simulink model "V2x_blockset"  (Simulink 7.6)
settings: Solver=ode45  StartTime=0.0  StopTime=10.0  RelTol=1e-3
undefined symbols (not defined in the file or in its folder): intmax, Newton, Raphson
libraries: simulink x53
(part 1 of 3)
settings Model: Creator=MarcinB  LastModifiedBy=pastora
settings SFSimCC: SimParseCustomCode=off

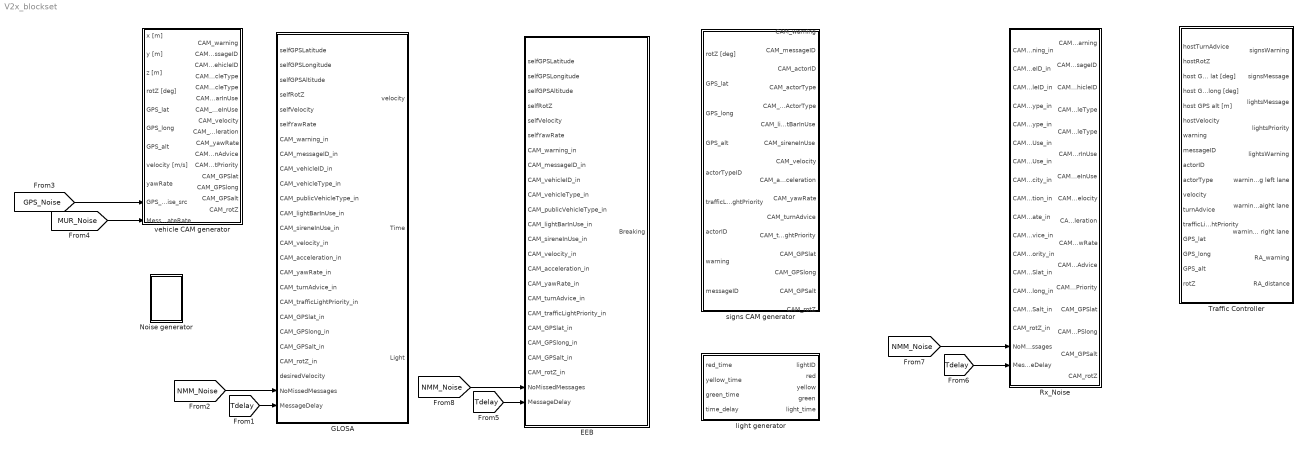
== system V2x_blockset ==
  EEB : Subsystem
  GLOSA : Subsystem
  Noise generator : Subsystem
  Rx_Noise : Subsystem
  Traffic Controller : Subsystem
  light generator : Subsystem
  signs CAM generator : Subsystem
  vehicle CAM generator : Subsystem
  wires:
  [NMM_Noise] -> GLOSA/24(NoMissedMessages)
  [Tdelay] -> GLOSA/25(MessageDelay)
  [MUR_Noise] -> vehicle CAM generator/11(MessageUpdateRate)
  [GPS_Noise] -> vehicle CAM generator/10(GPS_Noise_src)
  [NMM_Noise] -> Rx_Noise/17(NoMissedMessages)
  [Tdelay] -> Rx_Noise/18(MessageDelay)
  [NMM_Noise] -> EEB/23(NoMissedMessages)
  [Tdelay] -> EEB/24(MessageDelay)

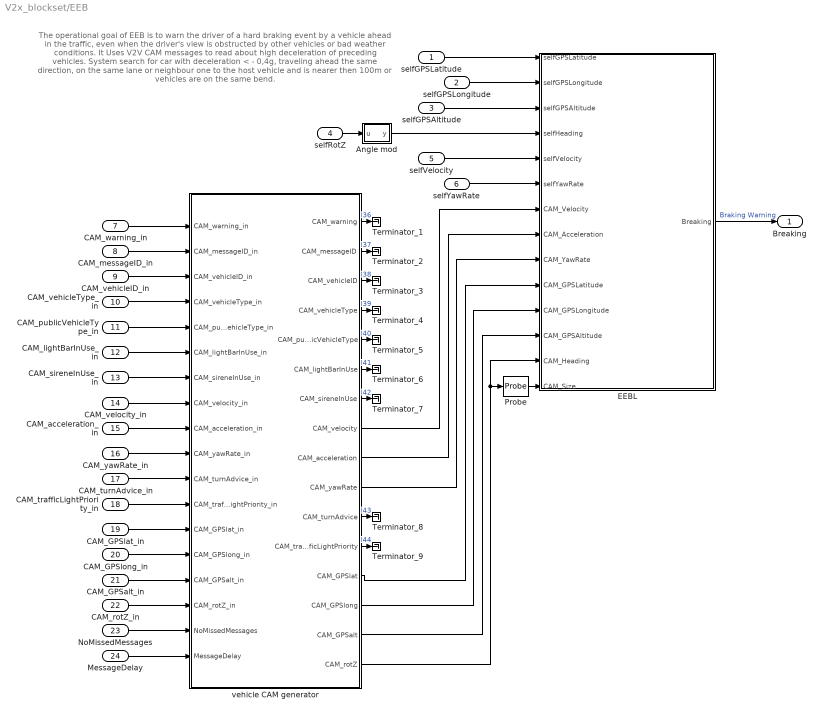
== system V2x_blockset/EEB ==
  note: The operational goal of EEB is to warn the driver of
      | a hard braking event by a vehicle ahead in the traffic,
      |  even when the driver's view is obstructed by
      |  other vehicles or bad weather conditions. It Uses V2V CAM
      | messages to read about high deceleration of preceding vehicles.
      | System search for car with deceleration < - 0,4g, traveling ahead
      |  the same direction, on the same lane or neighbour one to the host
      |  vehicle and is nearer then 100m or vehicles are on the same bend.
  selfGPSLatitude : Inport
  selfGPSLongitude : Inport  Port=2
  selfGPSAltitude : Inport  Port=3
  selfRotZ : Inport  Port=4
  selfVelocity : Inport  Port=5
  selfYawRate : Inport  Port=6
  CAM_warning_in : Inport  Port=7
  CAM_messageID_in : Inport  Port=8
  CAM_vehicleID_in : Inport  Port=9
  CAM_vehicleType_in : Inport  Port=10
  CAM_publicVehicleType_in : Inport  Port=11
  CAM_lightBarInUse_in : Inport  Port=12
  CAM_sireneInUse_in : Inport  Port=13
  CAM_velocity_in : Inport  Port=14
  CAM_acceleration_in : Inport  Port=15
  CAM_yawRate_in : Inport  Port=16
  CAM_turnAdvice_in : Inport  Port=17
  CAM_trafficLightPriority_in : Inport  Port=18
  CAM_GPSlat_in : Inport  Port=19
  CAM_GPSlong_in : Inport  Port=20
  CAM_GPSalt_in : Inport  Port=21
  CAM_rotZ_in : Inport  Port=22
  NoMissedMessages : Inport  Port=23
  MessageDelay : Inport  Port=24
  Angle mod : Stateflow chart  TreatAsAtomicUnit=on
  EEBL : Stateflow chart  TreatAsAtomicUnit=on
  Probe : Probe  ProbeWidth=off  ProbeSampleTime=off  ProbeComplexSignal=off  ProbeSignalDimensions=on
  Terminator_{1..9} (9 alike) : Terminator
  vehicle CAM generator : Subsystem
  Breaking : Outport
  wires:
  CAM_warning_in/1 -> vehicle CAM generator/1(CAM_warning_in)
  CAM_messageID_in/1 -> vehicle CAM generator/2(CAM_messageID_in)
  CAM_vehicleID_in/1 -> vehicle CAM generator/3(CAM_vehicleID_in)
  CAM_vehicleType_in/1 -> vehicle CAM generator/4(CAM_vehicleType_in)
  CAM_publicVehicleType_in/1 -> vehicle CAM generator/5(CAM_publicVehicleType_in)
  CAM_lightBarInUse_in/1 -> vehicle CAM generator/6(CAM_lightBarInUse_in)
  CAM_sireneInUse_in/1 -> vehicle CAM generator/7(CAM_sireneInUse_in)
  CAM_velocity_in/1 -> vehicle CAM generator/8(CAM_velocity_in)
  CAM_acceleration_in/1 -> vehicle CAM generator/9(CAM_acceleration_in)
  CAM_yawRate_in/1 -> vehicle CAM generator/10(CAM_yawRate_in)
  CAM_turnAdvice_in/1 -> vehicle CAM generator/11(CAM_turnAdvice_in)
  CAM_trafficLightPriority_in/1 -> vehicle CAM generator/12(CAM_trafficLightPriority_in)
  CAM_GPSlat_in/1 -> vehicle CAM generator/13(CAM_GPSlat_in)
  CAM_GPSlong_in/1 -> vehicle CAM generator/14(CAM_GPSlong_in)
  CAM_GPSalt_in/1 -> vehicle CAM generator/15(CAM_GPSalt_in)
  CAM_rotZ_in/1 -> vehicle CAM generator/16(CAM_rotZ_in)
  EEBL/1(Breaking) -> Breaking/1  "Braking Warning"
  selfGPSLatitude/1 -> EEBL/1(selfGPSLatitude)
  selfGPSLongitude/1 -> EEBL/2(selfGPSLongitude)
  selfGPSAltitude/1 -> EEBL/3(selfGPSAltitude)
  selfRotZ/1 -> Angle mod/1(u)
  selfVelocity/1 -> EEBL/5(selfVelocity)
  selfYawRate/1 -> EEBL/6(selfYawRate)
  NoMissedMessages/1 -> vehicle CAM generator/17(NoMissedMessages)
  MessageDelay/1 -> vehicle CAM generator/18(MessageDelay)
  vehicle CAM generator/8(CAM_velocity) -> EEBL/7(CAM_Velocity)
  vehicle CAM generator/16(CAM_rotZ) -> EEBL/13(CAM_Heading), Probe/1
  vehicle CAM generator/13(CAM_GPSlat) -> EEBL/10(CAM_GPSLatitude)
  vehicle CAM generator/14(CAM_GPSlong) -> EEBL/11(CAM_GPSLongitude)
  vehicle CAM generator/15(CAM_GPSalt) -> EEBL/12(CAM_GPSAltitude)
  vehicle CAM generator/10(CAM_yawRate) -> EEBL/9(CAM_YawRate)
  vehicle CAM generator/9(CAM_acceleration) -> EEBL/8(CAM_Acceleration)
  Angle mod/1(y) -> EEBL/4(selfHeading)
  Probe/1 -> EEBL/14(CAM_Size)
  vehicle CAM generator/1(CAM_warning) -> Terminator_1/1  "l36"
  vehicle CAM generator/2(CAM_messageID) -> Terminator_2/1  "l37"
  vehicle CAM generator/3(CAM_vehicleID) -> Terminator_3/1  "l38"
  vehicle CAM generator/4(CAM_vehicleType) -> Terminator_4/1  "l39"
  vehicle CAM generator/5(CAM_publicVehicleType) -> Terminator_5/1  "l40"
  vehicle CAM generator/6(CAM_lightBarInUse) -> Terminator_6/1  "l41"
  vehicle CAM generator/7(CAM_sireneInUse) -> Terminator_7/1  "l42"
  vehicle CAM generator/11(CAM_turnAdvice) -> Terminator_8/1  "l43"
  vehicle CAM generator/12(CAM_trafficLightPriority) -> Terminator_9/1  "l44"

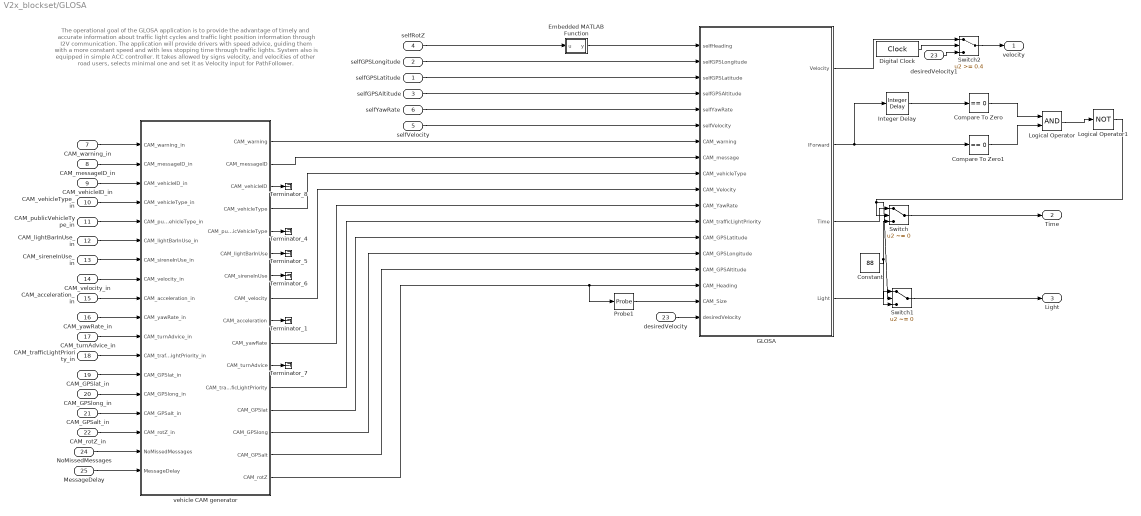
== system V2x_blockset/GLOSA ==
  note: The operational goal of the GLOSA application is to provide the advantage of
      |  timely and accurate information about traffic light cycles and
      |  traffic light position information through I2V communication.
      |  The application will provide drivers with speed advice, guiding them
      |  with a more constant speed and with less stopping time through traffic lights.
      |  System also is equipped in simple ACC controller.
      | It takes allowed by signs velocity, and velocities of other road users,
      |  selects minimal one and set it as Velocity input for PathFollower.
  selfGPSLatitude : Inport
  selfGPSLongitude : Inport  Port=2
  selfGPSAltitude : Inport  Port=3
  selfRotZ : Inport  Port=4
  selfVelocity : Inport  Port=5
  selfYawRate : Inport  Port=6
  CAM_warning_in : Inport  Port=7
  CAM_messageID_in : Inport  Port=8
  CAM_vehicleID_in : Inport  Port=9
  CAM_vehicleType_in : Inport  Port=10
  CAM_publicVehicleType_in : Inport  Port=11
  CAM_lightBarInUse_in : Inport  Port=12
  CAM_sireneInUse_in : Inport  Port=13
  CAM_velocity_in : Inport  Port=14
  CAM_acceleration_in : Inport  Port=15
  CAM_yawRate_in : Inport  Port=16
  CAM_turnAdvice_in : Inport  Port=17
  CAM_trafficLightPriority_in : Inport  Port=18
  CAM_GPSlat_in : Inport  Port=19
  CAM_GPSlong_in : Inport  Port=20
  CAM_GPSalt_in : Inport  Port=21
  CAM_rotZ_in : Inport  Port=22
  desiredVelocity : Inport  Port=23
  NoMissedMessages : Inport  Port=24
  MessageDelay : Inport  Port=25
  Compare To Zero : simulink/Logic and Bit Operations/Compare To Zero  SystemSampleTime=-1  relop===  LogicOutDataTypeMode=boolean
  Compare To Zero1 : simulink/Logic and Bit Operations/Compare To Zero  SystemSampleTime=-1  relop===  LogicOutDataTypeMode=boolean
  Constant : Constant  Value=88
  Digital Clock : DigitalClock
  Embedded MATLAB Function : Stateflow chart  TreatAsAtomicUnit=on
  GLOSA : Stateflow chart  TreatAsAtomicUnit=on
  Integer Delay : simulink/Discrete/Integer Delay  vinit=0.0  samptime=-1  NumDelays=5
  Logical Operator : Logic  AllPortsSameDT=off  OutDataTypeStr=boolean
  Logical Operator1 : Logic  Operator=NOT  AllPortsSameDT=off  OutDataTypeStr=boolean
  Probe1 : Probe  ProbeWidth=off  ProbeSampleTime=off  ProbeComplexSignal=off  ProbeSignalDimensions=on
  Switch : Switch  Criteria=u2 ~= 0
  Switch1 : Switch  Criteria=u2 ~= 0
  Switch2 : Switch  Threshold=0.4
  Terminator_{1,4..8} (6 alike) : Terminator
  desiredVelocity1 : InportShadow  Port=23
  vehicle CAM generator : Subsystem
  velocity : Outport
  Time : Outport  Port=2
  Light : Outport  Port=3
  wires:
  vehicle CAM generator/10(CAM_yawRate) -> GLOSA/11(CAM_YawRate)
  vehicle CAM generator/16(CAM_rotZ) -> GLOSA/16(CAM_Heading), Probe1/1
  vehicle CAM generator/15(CAM_GPSalt) -> GLOSA/15(CAM_GPSAltitude)
  vehicle CAM generator/13(CAM_GPSlat) -> GLOSA/13(CAM_GPSLatitude)
  vehicle CAM generator/14(CAM_GPSlong) -> GLOSA/14(CAM_GPSLongitude)
  vehicle CAM generator/8(CAM_velocity) -> GLOSA/10(CAM_Velocity)
  selfGPSLatitude/1 -> GLOSA/3(selfGPSLatitude)
  selfGPSLongitude/1 -> GLOSA/2(selfGPSLongitude)
  selfGPSAltitude/1 -> GLOSA/4(selfGPSAltitude)
  selfRotZ/1 -> Embedded MATLAB Function/1(u)
  selfVelocity/1 -> GLOSA/6(selfVelocity)
  selfYawRate/1 -> GLOSA/5(selfYawRate)
  CAM_warning_in/1 -> vehicle CAM generator/1(CAM_warning_in)
  CAM_messageID_in/1 -> vehicle CAM generator/2(CAM_messageID_in)
  CAM_vehicleID_in/1 -> vehicle CAM generator/3(CAM_vehicleID_in)
  CAM_vehicleType_in/1 -> vehicle CAM generator/4(CAM_vehicleType_in)
  CAM_publicVehicleType_in/1 -> vehicle CAM generator/5(CAM_publicVehicleType_in)
  CAM_lightBarInUse_in/1 -> vehicle CAM generator/6(CAM_lightBarInUse_in)
  CAM_sireneInUse_in/1 -> vehicle CAM generator/7(CAM_sireneInUse_in)
  CAM_velocity_in/1 -> vehicle CAM generator/8(CAM_velocity_in)
  CAM_acceleration_in/1 -> vehicle CAM generator/9(CAM_acceleration_in)
  CAM_yawRate_in/1 -> vehicle CAM generator/10(CAM_yawRate_in)
  CAM_turnAdvice_in/1 -> vehicle CAM generator/11(CAM_turnAdvice_in)
  CAM_trafficLightPriority_in/1 -> vehicle CAM generator/12(CAM_trafficLightPriority_in)
  CAM_GPSlat_in/1 -> vehicle CAM generator/13(CAM_GPSlat_in)
  CAM_GPSlong_in/1 -> vehicle CAM generator/14(CAM_GPSlong_in)
  CAM_GPSalt_in/1 -> vehicle CAM generator/15(CAM_GPSalt_in)
  CAM_rotZ_in/1 -> vehicle CAM generator/16(CAM_rotZ_in)
  vehicle CAM generator/1(CAM_warning) -> GLOSA/7(CAM_warning)
  vehicle CAM generator/2(CAM_messageID) -> GLOSA/8(CAM_message)
  vehicle CAM generator/4(CAM_vehicleType) -> GLOSA/9(CAM_vehicleType)
  vehicle CAM generator/5(CAM_publicVehicleType) -> Terminator_4/1
  vehicle CAM generator/6(CAM_lightBarInUse) -> Terminator_5/1
  vehicle CAM generator/7(CAM_sireneInUse) -> Terminator_6/1
  vehicle CAM generator/11(CAM_turnAdvice) -> Terminator_7/1
  vehicle CAM generator/12(CAM_trafficLightPriority) -> GLOSA/12(CAM_trafficLightPriority)
  desiredVelocity/1 -> GLOSA/18(desiredVelocity)
  vehicle CAM generator/3(CAM_vehicleID) -> Terminator_8/1
  Embedded MATLAB Function/1(y) -> GLOSA/1(selfHeading)
  NoMissedMessages/1 -> vehicle CAM generator/17(NoMissedMessages)
  MessageDelay/1 -> vehicle CAM generator/18(MessageDelay)
  Probe1/1 -> GLOSA/17(CAM_Size)
  vehicle CAM generator/9(CAM_acceleration) -> Terminator_1/1
  GLOSA/3(Time) -> Switch/1
  GLOSA/4(Light) -> Switch1/1
  GLOSA/2(lForward) -> Integer Delay/1, Compare To Zero1/1
  Constant/1 -> Switch/3, Switch1/3
  Switch1/1 -> Light/1
  Switch/1 -> Time/1
  Integer Delay/1 -> Compare To Zero/1
  Compare To Zero/1 -> Logical Operator/1
  Compare To Zero1/1 -> Logical Operator/2
  Logical Operator/1 -> Logical Operator1/1
  Logical Operator1/1 -> Switch/2, Switch1/2
  Digital Clock/1 -> Switch2/2
  Switch2/1 -> velocity/1
  GLOSA/1(Velocity) -> Switch2/1
  desiredVelocity1/1 -> Switch2/3

== system V2x_blockset/Noise generator ==
  DISPLAY : M-S-Function  FunctionName=msfcn_V2X_PlotSpeed
  Scope1 : Scope  NumInputPorts=4
      settings: YMin=-5~-5~-5~-5  YMax=5~5~5~5
  tag scope: GPS_Noise=global, MUR_Noise=global, NMM_Noise=global, Tdelay=global
  wires:
  DISPLAY/1 -> Scope1/1, [GPS_Noise]
  DISPLAY/2 -> Scope1/2, [MUR_Noise]
  DISPLAY/3 -> Scope1/3, [NMM_Noise]
  DISPLAY/4 -> Scope1/4, [Tdelay]

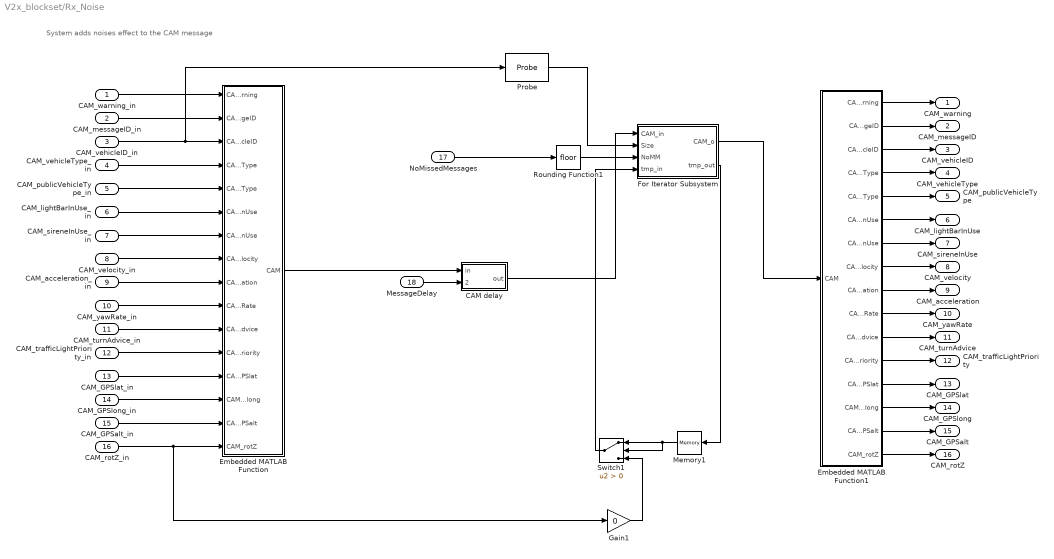
== system V2x_blockset/Rx_Noise ==
  note: System adds noises effect to the CAM message
  CAM_warning_in : Inport
  CAM_messageID_in : Inport  Port=2
  CAM_vehicleID_in : Inport  Port=3
  CAM_vehicleType_in : Inport  Port=4
  CAM_publicVehicleType_in : Inport  Port=5
  CAM_lightBarInUse_in : Inport  Port=6
  CAM_sireneInUse_in : Inport  Port=7
  CAM_velocity_in : Inport  Port=8
  CAM_acceleration_in : Inport  Port=9
  CAM_yawRate_in : Inport  Port=10
  CAM_turnAdvice_in : Inport  Port=11
  CAM_trafficLightPriority_in : Inport  Port=12
  CAM_GPSlat_in : Inport  Port=13
  CAM_GPSlong_in : Inport  Port=14
  CAM_GPSalt_in : Inport  Port=15
  CAM_rotZ_in : Inport  Port=16
  NoMissedMessages : Inport  Port=17
  MessageDelay : Inport  Port=18
  CAM delay : Subsystem
  Embedded MATLAB Function : Stateflow chart  TreatAsAtomicUnit=on
  Embedded MATLAB Function1 : Stateflow chart  TreatAsAtomicUnit=on
  For Iterator Subsystem : Subsystem  TreatAsAtomicUnit=on
  Gain1 : Gain  Gain=0
  Memory1 : Memory
  Probe : Probe  ProbeWidth=off  ProbeSampleTime=off  ProbeComplexSignal=off  ProbeSignalDimensions=on
  Rounding Function1 : Rounding
  Switch1 : Switch  Criteria=u2 > Threshold
  CAM_warning : Outport
  CAM_messageID : Outport  Port=2
  CAM_vehicleID : Outport  Port=3
  CAM_vehicleType : Outport  Port=4
  CAM_publicVehicleType : Outport  Port=5
  CAM_lightBarInUse : Outport  Port=6
  CAM_sireneInUse : Outport  Port=7
  CAM_velocity : Outport  Port=8
  CAM_acceleration : Outport  Port=9
  CAM_yawRate : Outport  Port=10
  CAM_turnAdvice : Outport  Port=11
  CAM_trafficLightPriority : Outport  Port=12
  CAM_GPSlat : Outport  Port=13
  CAM_GPSlong : Outport  Port=14
  CAM_GPSalt : Outport  Port=15
  CAM_rotZ : Outport  Port=16
  wires:
  Embedded MATLAB Function1/16(CAM_rotZ) -> CAM_rotZ/1
  Embedded MATLAB Function1/15(CAM_GPSalt) -> CAM_GPSalt/1
  Embedded MATLAB Function1/14(CAM_GPSlong) -> CAM_GPSlong/1
  Embedded MATLAB Function1/13(CAM_GPSlat) -> CAM_GPSlat/1
  Embedded MATLAB Function1/12(CAM_trafficLightPriority) -> CAM_trafficLightPriority/1
  Embedded MATLAB Function1/11(CAM_turnAdvice) -> CAM_turnAdvice/1
  Embedded MATLAB Function1/10(CAM_yawRate) -> CAM_yawRate/1
  Embedded MATLAB Function1/9(CAM_acceleration) -> CAM_acceleration/1
  Embedded MATLAB Function1/8(CAM_velocity) -> CAM_velocity/1
  Embedded MATLAB Function1/7(CAM_sireneInUse) -> CAM_sireneInUse/1
  Embedded MATLAB Function1/6(CAM_lightBarInUse) -> CAM_lightBarInUse/1
  Embedded MATLAB Function1/5(CAM_publicVehicleType) -> CAM_publicVehicleType/1
  Embedded MATLAB Function1/4(CAM_vehicleType) -> CAM_vehicleType/1
  Embedded MATLAB Function1/3(CAM_vehicleID) -> CAM_vehicleID/1
  Embedded MATLAB Function1/2(CAM_messageID) -> CAM_messageID/1
  Embedded MATLAB Function1/1(CAM_warning) -> CAM_warning/1
  CAM_warning_in/1 -> Embedded MATLAB Function/1(CAM_warning)
  CAM_messageID_in/1 -> Embedded MATLAB Function/2(CAM_messageID)
  CAM_vehicleID_in/1 -> Embedded MATLAB Function/3(CAM_vehicleID), Probe/1
  CAM_vehicleType_in/1 -> Embedded MATLAB Function/4(CAM_vehicleType)
  CAM_publicVehicleType_in/1 -> Embedded MATLAB Function/5(CAM_publicVehicleType)
  CAM_lightBarInUse_in/1 -> Embedded MATLAB Function/6(CAM_lightBarInUse)
  CAM_sireneInUse_in/1 -> Embedded MATLAB Function/7(CAM_sireneInUse)
  CAM_velocity_in/1 -> Embedded MATLAB Function/8(CAM_velocity)
  CAM_acceleration_in/1 -> Embedded MATLAB Function/9(CAM_acceleration)
  CAM_yawRate_in/1 -> Embedded MATLAB Function/10(CAM_yawRate)
  CAM_turnAdvice_in/1 -> Embedded MATLAB Function/11(CAM_turnAdvice)
  CAM_trafficLightPriority_in/1 -> Embedded MATLAB Function/12(CAM_trafficLightPriority)
  CAM_GPSlat_in/1 -> Embedded MATLAB Function/13(CAM_GPSlat)
  CAM_GPSlong_in/1 -> Embedded MATLAB Function/14(CAM_GPSlong)
  CAM_GPSalt_in/1 -> Embedded MATLAB Function/15(CAM_GPSalt)
  CAM_rotZ_in/1 -> Embedded MATLAB Function/16(CAM_rotZ), Gain1/1
  Probe/1 -> For Iterator Subsystem/2(Size)
  Embedded MATLAB Function/1(CAM) -> CAM delay/1(in)
  MessageDelay/1 -> CAM delay/2(Tdelay)
  CAM delay/1(out) -> For Iterator Subsystem/1(CAM_in)
  For Iterator Subsystem/2(tmp_out) -> Memory1/1
  Memory1/1 -> Switch1/2, Switch1/1
  NoMissedMessages/1 -> Rounding Function1/1
  Rounding Function1/1 -> For Iterator Subsystem/3(NoMM)
  Gain1/1 -> Switch1/3
  Switch1/1 -> For Iterator Subsystem/4(tmp_in)
  For Iterator Subsystem/1(CAM_o) -> Embedded MATLAB Function1/1(CAM)

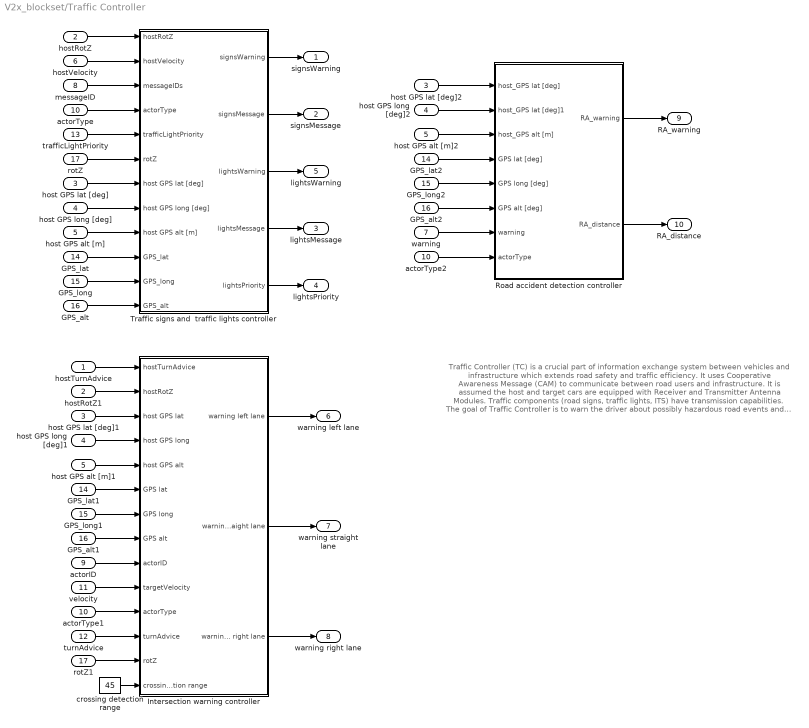
== system V2x_blockset/Traffic Controller ==
  note: Traffic Controller (TC) is a crucial part of information exchange system between
      |  vehicles and infrastructure which extends road safety and traffic efficiency.
      |  It uses Cooperative Awareness Message (CAM) to communicate between road users and infrastructure.
      |  It is assumed the host and target cars are equipped with Receiver and Transmitter Antenna Modules.
      |  Traffic components (road signs, traffic lights, ITS) have transmission capabilities.
      | The goal of Traffic Controller is to warn the driver about possibly hazardous road events and about breaking traffic rules.
  hostTurnAdvice : Inport
  hostRotZ : Inport  Port=2
  host GPS lat [deg] : Inport  Port=3
  host GPS long [deg] : Inport  Port=4
  host GPS alt [m] : Inport  Port=5
  hostVelocity : Inport  Port=6
  warning : Inport  Port=7
  messageID : Inport  Port=8
  actorID : Inport  Port=9
  actorType : Inport  Port=10
  velocity : Inport  Port=11
  turnAdvice : Inport  Port=12
  trafficLightPriority : Inport  Port=13
  GPS_lat : Inport  Port=14
  GPS_long : Inport  Port=15
  GPS_alt : Inport  Port=16
  rotZ : Inport  Port=17
  GPS_alt1 : InportShadow  Port=16
  GPS_alt2 : InportShadow  Port=16
  GPS_lat1 : InportShadow  Port=14
  GPS_lat2 : InportShadow  Port=14
  GPS_long1 : InportShadow  Port=15
  GPS_long2 : InportShadow  Port=15
  Intersection warning controller : Subsystem
  Road accident detection controller : Subsystem
  Traffic signs and  traffic lights controller : Subsystem
  actorType1 : InportShadow  Port=10
  actorType2 : InportShadow  Port=10
  crossing detection range : Constant  Value=45
  host GPS alt [m]1 : InportShadow  Port=5
  host GPS alt [m]2 : InportShadow  Port=5
  host GPS lat [deg]1 : InportShadow  Port=3
  host GPS lat [deg]2 : InportShadow  Port=3
  host GPS long [deg]1 : InportShadow  Port=4
  host GPS long [deg]2 : InportShadow  Port=4
  hostRotZ1 : InportShadow  Port=2
  rotZ1 : InportShadow  Port=17
  signsWarning : Outport
  signsMessage : Outport  Port=2
  lightsMessage : Outport  Port=3
  lightsPriority : Outport  Port=4
  lightsWarning : Outport  Port=5
  warning left lane : Outport  Port=6
  warning straight lane : Outport  Port=7
  warning right lane : Outport  Port=8
  RA_warning : Outport  Port=9
  RA_distance : Outport  Port=10
  wires:
  hostRotZ/1 -> Traffic signs and  traffic lights controller/1(hostRotZ)
  hostVelocity/1 -> Traffic signs and  traffic lights controller/2(hostVelocity)
  messageID/1 -> Traffic signs and  traffic lights controller/3(messageIDs)
  actorType/1 -> Traffic signs and  traffic lights controller/4(actorType)
  rotZ/1 -> Traffic signs and  traffic lights controller/6(rotZ)
  trafficLightPriority/1 -> Traffic signs and  traffic lights controller/5(trafficLightPriority)
  Traffic signs and  traffic lights controller/2(signsMessage) -> signsMessage/1
  Traffic signs and  traffic lights controller/1(signsWarning) -> signsWarning/1
  Traffic signs and  traffic lights controller/3(lightsWarning) -> lightsWarning/1
  Traffic signs and  traffic lights controller/4(lightsMessage) -> lightsMessage/1
  Traffic signs and  traffic lights controller/5(lightsPriority) -> lightsPriority/1
  host GPS lat [deg]/1 -> Traffic signs and  traffic lights controller/7(host GPS lat [deg])
  host GPS long [deg]/1 -> Traffic signs and  traffic lights controller/8(host GPS long [deg])
  host GPS alt [m]/1 -> Traffic signs and  traffic lights controller/9(host GPS alt [m])
  GPS_lat/1 -> Traffic signs and  traffic lights controller/10(GPS_lat)
  GPS_long/1 -> Traffic signs and  traffic lights controller/11(GPS_long)
  GPS_alt/1 -> Traffic signs and  traffic lights controller/12(GPS_alt)
  Intersection warning controller/1(warning left lane) -> warning left lane/1
  Intersection warning controller/2(warning straight lane) -> warning straight lane/1
  Intersection warning controller/3(warning right lane) -> warning right lane/1
  hostTurnAdvice/1 -> Intersection warning controller/1(hostTurnAdvice)
  hostRotZ1/1 -> Intersection warning controller/2(hostRotZ)
  host GPS lat [deg]1/1 -> Intersection warning controller/3(host GPS lat)
  host GPS long [deg]1/1 -> Intersection warning controller/4(host GPS long)
  host GPS alt [m]1/1 -> Intersection warning controller/5(host GPS alt)
  GPS_lat1/1 -> Intersection warning controller/6(GPS lat)
  GPS_long1/1 -> Intersection warning controller/7(GPS long)
  GPS_alt1/1 -> Intersection warning controller/8(GPS alt)
  actorID/1 -> Intersection warning controller/9(actorID)
  actorType1/1 -> Intersection warning controller/11(actorType)
  turnAdvice/1 -> Intersection warning controller/12(turnAdvice)
  rotZ1/1 -> Intersection warning controller/13(rotZ)
  crossing detection range/1 -> Intersection warning controller/14(crossing detection range)
  velocity/1 -> Intersection warning controller/10(targetVelocity)
  Road accident detection controller/1(RA_warning) -> RA_warning/1
  Road accident detection controller/2(RA_distance) -> RA_distance/1
  host GPS lat [deg]2/1 -> Road accident detection controller/1(host_GPS lat [deg])
  host GPS long [deg]2/1 -> Road accident detection controller/2(host_GPS lat [deg]1)
  host GPS alt [m]2/1 -> Road accident detection controller/3(host_GPS alt [m])
  GPS_lat2/1 -> Road accident detection controller/4(GPS lat [deg])
  GPS_long2/1 -> Road accident detection controller/5(GPS long [deg])
  GPS_alt2/1 -> Road accident detection controller/6(GPS alt [deg])
  warning/1 -> Road accident detection controller/7(warning)
  actorType2/1 -> Road accident detection controller/8(actorType)

== system V2x_blockset/light generator ==
  red_time : Inport
  yellow_time : Inport  Port=2
  green_time : Inport  Port=3
  time_delay : Inport  Port=4
  Clock : Clock
      settings: Decimation=10
  Lights generator : Stateflow chart  TreatAsAtomicUnit=on
  Memory2 : Memory
  lightID : Outport
  red : Outport  Port=2
  yellow : Outport  Port=3
  green : Outport  Port=4
  light_time : Outport  Port=5
  wires:
  Clock/1 -> Lights generator/4(time)
  Lights generator/6(last_time_out) -> Memory2/1
  Memory2/1 -> Lights generator/6(last_time)
  red_time/1 -> Lights generator/1(red_time)
  yellow_time/1 -> Lights generator/2(yellow_time)
  green_time/1 -> Lights generator/3(green_time)
  time_delay/1 -> Lights generator/5(time_delay)
  Lights generator/1(lightID) -> lightID/1
  Lights generator/2(red) -> red/1
  Lights generator/3(yellow) -> yellow/1
  Lights generator/4(green) -> green/1
  Lights generator/5(light_time) -> light_time/1

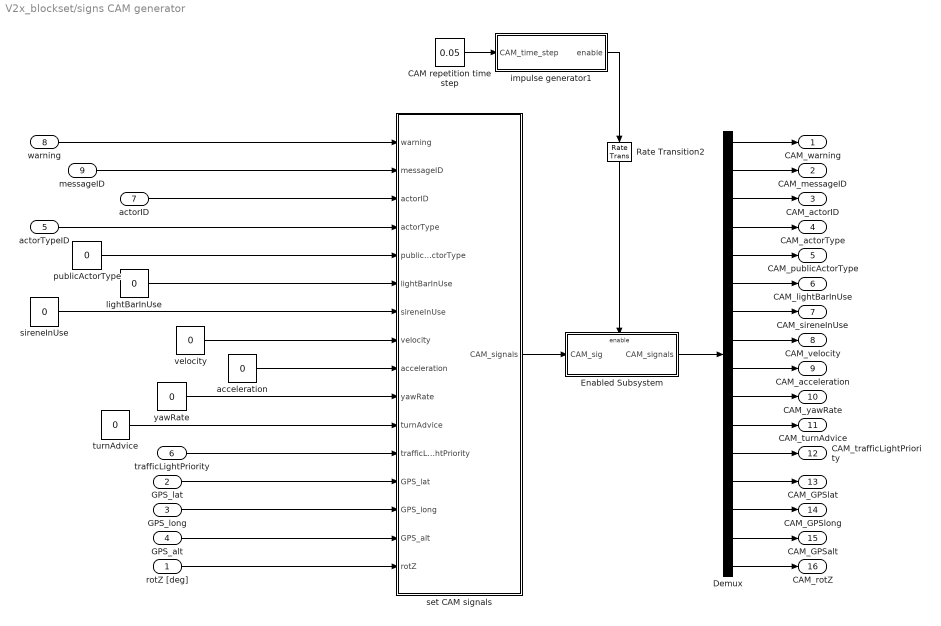
== system V2x_blockset/signs CAM generator ==
  rotZ [deg] : Inport
  GPS_lat : Inport  Port=2
  GPS_long : Inport  Port=3
  GPS_alt : Inport  Port=4
  actorTypeID : Inport  Port=5
  trafficLightPriority : Inport  Port=6
  actorID : Inport  Port=7
  warning : Inport  Port=8
  messageID : Inport  Port=9
  CAM repetition time step : Constant  Value=0.05
  Demux : Demux  Outputs=16
  Enabled Subsystem : Subsystem  TreatAsAtomicUnit=on
  Rate Transition2 : RateTransition  Integrity=off  OutPortSampleTimeOpt=Inherit
  acceleration : Constant  Value=0
  impulse generator1 : Subsystem
  lightBarInUse : Constant  Value=0
  publicActorType : Constant  Value=0
  set CAM signals : Subsystem
  sireneInUse : Constant  Value=0
  turnAdvice : Constant  Value=0
  velocity : Constant  Value=0
  yawRate : Constant  Value=0
  CAM_warning : Outport
  CAM_messageID : Outport  Port=2
  CAM_actorID : Outport  Port=3
  CAM_actorType : Outport  Port=4
  CAM_publicActorType : Outport  Port=5
  CAM_lightBarInUse : Outport  Port=6
  CAM_sireneInUse : Outport  Port=7
  CAM_velocity : Outport  Port=8
  CAM_acceleration : Outport  Port=9
  CAM_yawRate : Outport  Port=10
  CAM_turnAdvice : Outport  Port=11
  CAM_trafficLightPriority : Outport  Port=12
  CAM_GPSlat : Outport  Port=13
  CAM_GPSlong : Outport  Port=14
  CAM_GPSalt : Outport  Port=15
  CAM_rotZ : Outport  Port=16
  wires:
  CAM repetition time step/1 -> impulse generator1/1(CAM_time_step)
  impulse generator1/1(enable) -> Rate Transition2/1
  warning/1 -> set CAM signals/1(warning)
  messageID/1 -> set CAM signals/2(messageID)
  actorID/1 -> set CAM signals/3(actorID)
  actorTypeID/1 -> set CAM signals/4(actorType)
  publicActorType/1 -> set CAM signals/5(publicActorType)
  lightBarInUse/1 -> set CAM signals/6(lightBarInUse)
  sireneInUse/1 -> set CAM signals/7(sireneInUse)
  yawRate/1 -> set CAM signals/10(yawRate)
  turnAdvice/1 -> set CAM signals/11(turnAdvice)
  trafficLightPriority/1 -> set CAM signals/12(trafficLightPriority)
  GPS_lat/1 -> set CAM signals/13(GPS_lat)
  GPS_long/1 -> set CAM signals/14(GPS_long)
  GPS_alt/1 -> set CAM signals/15(GPS_alt)
  rotZ [deg]/1 -> set CAM signals/16(rotZ)
  set CAM signals/1(CAM_signals) -> Enabled Subsystem/1(CAM_sig)
  Rate Transition2/1 -> Enabled Subsystem/Enable
  Enabled Subsystem/1(CAM_signals) -> Demux/1
  Demux/1 -> CAM_warning/1
  Demux/2 -> CAM_messageID/1
  Demux/3 -> CAM_actorID/1
  Demux/4 -> CAM_actorType/1
  Demux/5 -> CAM_publicActorType/1
  Demux/6 -> CAM_lightBarInUse/1
  Demux/7 -> CAM_sireneInUse/1
  Demux/8 -> CAM_velocity/1
  Demux/9 -> CAM_acceleration/1
  Demux/10 -> CAM_yawRate/1
  Demux/11 -> CAM_turnAdvice/1
  Demux/12 -> CAM_trafficLightPriority/1
  Demux/13 -> CAM_GPSlat/1
  Demux/14 -> CAM_GPSlong/1
  Demux/15 -> CAM_GPSalt/1
  Demux/16 -> CAM_rotZ/1
  velocity/1 -> set CAM signals/8(velocity)
  acceleration/1 -> set CAM signals/9(acceleration)

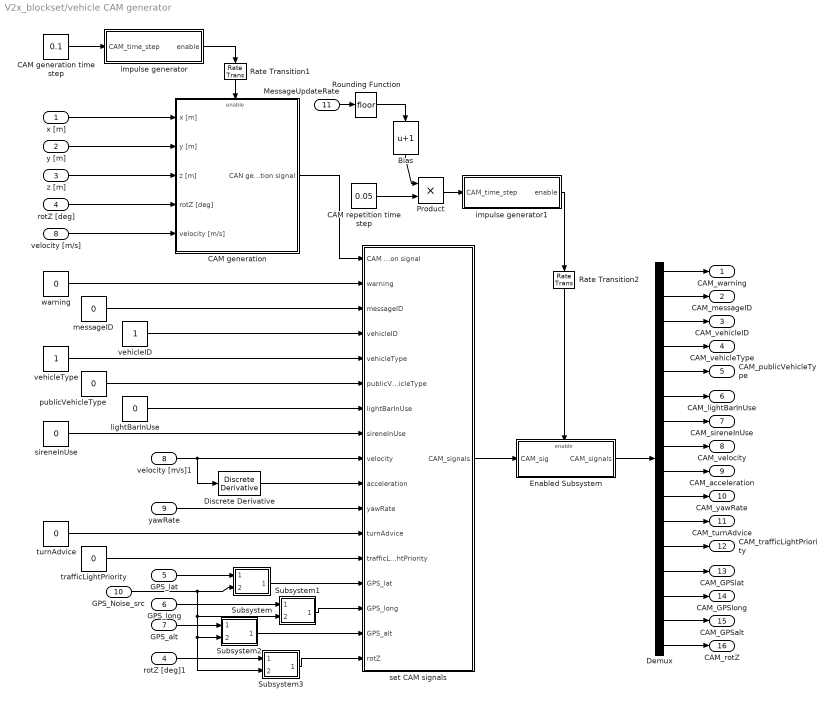
== system V2x_blockset/vehicle CAM generator ==
  x [m] : Inport
  y [m] : Inport  Port=2
  z [m] : Inport  Port=3
  rotZ [deg] : Inport  Port=4
  GPS_lat : Inport  Port=5
  GPS_long : Inport  Port=6
  GPS_alt : Inport  Port=7
  velocity [m/s] : Inport  Port=8
  yawRate : Inport  Port=9
  GPS_Noise_src : Inport  Port=10
  MessageUpdateRate : Inport  Port=11
  Bias : Bias  Bias=1
  CAM generation : Subsystem  TreatAsAtomicUnit=on
  CAM generation time step : Constant  Value=0.1
  CAM repetition time step : Constant  Value=0.05
  Demux : Demux  Outputs=16
  Discrete Derivative : simulink/Discrete/Discrete Derivative  SystemSampleTime=-1  gainval=1.0  ICPrevScaledInput=0.0  OutMin=[]  OutMax=[]  OutDataType=fixdt(1, 16)  OutScaling=2^-10  DoSatur=off
  Enabled Subsystem : Subsystem  TreatAsAtomicUnit=on
  Product : Product  RndMeth=Zero
  Rate Transition1 : RateTransition  Integrity=off  OutPortSampleTimeOpt=Inherit
  Rate Transition2 : RateTransition  Integrity=off  OutPortSampleTimeOpt=Inherit
  Rounding Function : Rounding
  Subsystem : Subsystem
  Subsystem1 : Subsystem
  Subsystem2 : Subsystem
  Subsystem3 : Subsystem
  impulse generator : Subsystem
  impulse generator1 : Subsystem
  lightBarInUse : Constant  Value=0
  messageID : Constant  Value=0
  publicVehicleType : Constant  Value=0
  rotZ [deg]1 : InportShadow  Port=4
  set CAM signals : Subsystem
  sireneInUse : Constant  Value=0
  trafficLightPriority : Constant  Value=0
  turnAdvice : Constant  Value=0
  vehicleID : Constant
  vehicleType : Constant
  velocity [m/s]1 : InportShadow  Port=8
  warning : Constant  Value=0
  CAM_warning : Outport
  CAM_messageID : Outport  Port=2
  CAM_vehicleID : Outport  Port=3
  CAM_vehicleType : Outport  Port=4
  CAM_publicVehicleType : Outport  Port=5
  CAM_lightBarInUse : Outport  Port=6
  CAM_sireneInUse : Outport  Port=7
  CAM_velocity : Outport  Port=8
  CAM_acceleration : Outport  Port=9
  CAM_yawRate : Outport  Port=10
  CAM_turnAdvice : Outport  Port=11
  CAM_trafficLightPriority : Outport  Port=12
  CAM_GPSlat : Outport  Port=13
  CAM_GPSlong : Outport  Port=14
  CAM_GPSalt : Outport  Port=15
  CAM_rotZ : Outport  Port=16
  wires:
  CAM generation time step/1 -> impulse generator/1(CAM_time_step)
  impulse generator1/1(enable) -> Rate Transition2/1
  warning/1 -> set CAM signals/2(warning)
  messageID/1 -> set CAM signals/3(messageID)
  vehicleID/1 -> set CAM signals/4(vehicleID)
  vehicleType/1 -> set CAM signals/5(vehicleType)
  publicVehicleType/1 -> set CAM signals/6(publicVehicleType)
  lightBarInUse/1 -> set CAM signals/7(lightBarInUse)
  sireneInUse/1 -> set CAM signals/8(sireneInUse)
  velocity [m/s]1/1 -> Discrete Derivative/1, set CAM signals/9(velocity)
  Discrete Derivative/1 -> set CAM signals/10(acceleration)
  yawRate/1 -> set CAM signals/11(yawRate)
  turnAdvice/1 -> set CAM signals/12(turnAdvice)
  trafficLightPriority/1 -> set CAM signals/13(trafficLightPriority)
  GPS_lat/1 -> Subsystem/1(In1)
  GPS_long/1 -> Subsystem1/1(In1)
  GPS_alt/1 -> Subsystem2/1(In1)
  rotZ [deg]1/1 -> Subsystem3/1(In1)
  CAM generation/1(CAN generation signal) -> set CAM signals/1(CAM generation signal)
  x [m]/1 -> CAM generation/1(x [m])
  y [m]/1 -> CAM generation/2(y [m])
  z [m]/1 -> CAM generation/3(z [m])
  rotZ [deg]/1 -> CAM generation/4(rotZ [deg])
  velocity [m/s]/1 -> CAM generation/5(velocity [m/s])
  impulse generator/1(enable) -> Rate Transition1/1
  Rate Transition1/1 -> CAM generation/Enable
  set CAM signals/1(CAM_signals) -> Enabled Subsystem/1(CAM_sig)
  Rate Transition2/1 -> Enabled Subsystem/Enable
  Enabled Subsystem/1(CAM_signals) -> Demux/1
  Demux/1 -> CAM_warning/1
  Demux/2 -> CAM_messageID/1
  Demux/3 -> CAM_vehicleID/1
  Demux/4 -> CAM_vehicleType/1
  Demux/5 -> CAM_publicVehicleType/1
  Demux/6 -> CAM_lightBarInUse/1
  Demux/7 -> CAM_sireneInUse/1
  Demux/8 -> CAM_velocity/1
  Demux/9 -> CAM_acceleration/1
  Demux/10 -> CAM_yawRate/1
  Demux/11 -> CAM_turnAdvice/1
  Demux/12 -> CAM_trafficLightPriority/1
  Demux/13 -> CAM_GPSlat/1
  Demux/14 -> CAM_GPSlong/1
  Demux/15 -> CAM_GPSalt/1
  Demux/16 -> CAM_rotZ/1
  Subsystem/1(Out1) -> set CAM signals/14(GPS_lat)
  Subsystem1/1(Out1) -> set CAM signals/15(GPS_long)
  Subsystem2/1(Out1) -> set CAM signals/16(GPS_alt)
  Subsystem3/1(Out1) -> set CAM signals/17(rotZ)
  Product/1 -> impulse generator1/1(CAM_time_step)
  CAM repetition time step/1 -> Product/2
  MessageUpdateRate/1 -> Rounding Function/1
  Rounding Function/1 -> Bias/1
  Bias/1 -> Product/1
  GPS_Noise_src/1 -> Subsystem/2(GPS_Noise_src), Subsystem1/2(GPS_Noise_src), Subsystem2/2(GPS_Noise_src), Subsystem3/2(GPS_Noise_src)

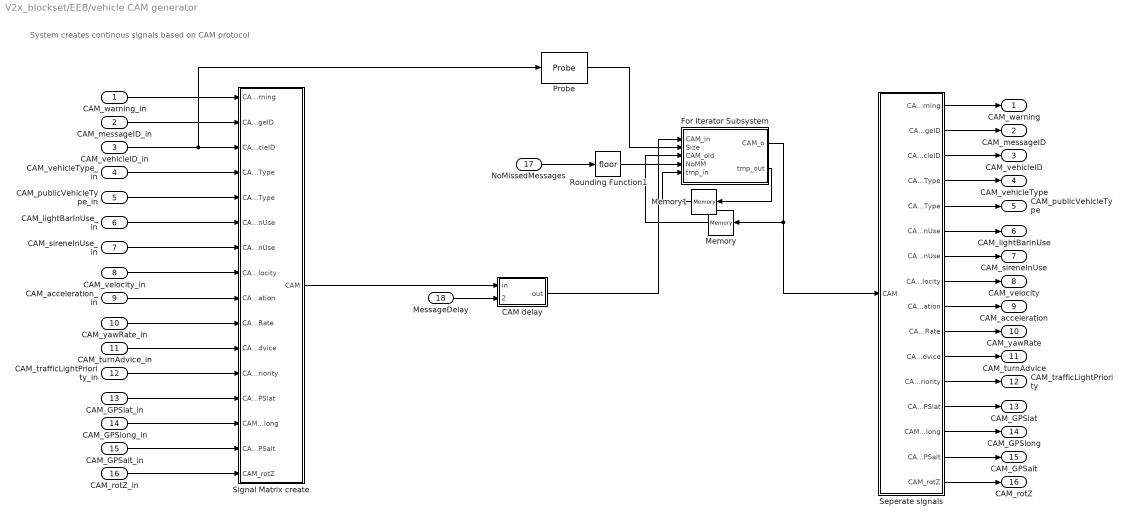
== system V2x_blockset/EEB/vehicle CAM generator ==
  note: System creates continous signals based on CAM protocol
  CAM_warning_in : Inport
  CAM_messageID_in : Inport  Port=2
  CAM_vehicleID_in : Inport  Port=3
  CAM_vehicleType_in : Inport  Port=4
  CAM_publicVehicleType_in : Inport  Port=5
  CAM_lightBarInUse_in : Inport  Port=6
  CAM_sireneInUse_in : Inport  Port=7
  CAM_velocity_in : Inport  Port=8
  CAM_acceleration_in : Inport  Port=9
  CAM_yawRate_in : Inport  Port=10
  CAM_turnAdvice_in : Inport  Port=11
  CAM_trafficLightPriority_in : Inport  Port=12
  CAM_GPSlat_in : Inport  Port=13
  CAM_GPSlong_in : Inport  Port=14
  CAM_GPSalt_in : Inport  Port=15
  CAM_rotZ_in : Inport  Port=16
  NoMissedMessages : Inport  Port=17
  MessageDelay : Inport  Port=18
  CAM delay : Subsystem
  For Iterator Subsystem : Subsystem  TreatAsAtomicUnit=on
  Memory : Memory
  Memory1 : Memory
  Probe : Probe  ProbeWidth=off  ProbeSampleTime=off  ProbeComplexSignal=off  ProbeSignalDimensions=on
  Rounding Function1 : Rounding
  Seperate signals : Stateflow chart  TreatAsAtomicUnit=on
  Signal Matrix create : Stateflow chart  TreatAsAtomicUnit=on
  CAM_warning : Outport
  CAM_messageID : Outport  Port=2
  CAM_vehicleID : Outport  Port=3
  CAM_vehicleType : Outport  Port=4
  CAM_publicVehicleType : Outport  Port=5
  CAM_lightBarInUse : Outport  Port=6
  CAM_sireneInUse : Outport  Port=7
  CAM_velocity : Outport  Port=8
  CAM_acceleration : Outport  Port=9
  CAM_yawRate : Outport  Port=10
  CAM_turnAdvice : Outport  Port=11
  CAM_trafficLightPriority : Outport  Port=12
  CAM_GPSlat : Outport  Port=13
  CAM_GPSlong : Outport  Port=14
  CAM_GPSalt : Outport  Port=15
  CAM_rotZ : Outport  Port=16
  wires:
  Seperate signals/16(CAM_rotZ) -> CAM_rotZ/1
  Seperate signals/15(CAM_GPSalt) -> CAM_GPSalt/1
  Seperate signals/14(CAM_GPSlong) -> CAM_GPSlong/1
  Seperate signals/13(CAM_GPSlat) -> CAM_GPSlat/1
  Seperate signals/12(CAM_trafficLightPriority) -> CAM_trafficLightPriority/1
  Seperate signals/11(CAM_turnAdvice) -> CAM_turnAdvice/1
  Seperate signals/10(CAM_yawRate) -> CAM_yawRate/1
  Seperate signals/9(CAM_acceleration) -> CAM_acceleration/1
  Seperate signals/8(CAM_velocity) -> CAM_velocity/1
  Seperate signals/7(CAM_sireneInUse) -> CAM_sireneInUse/1
  Seperate signals/6(CAM_lightBarInUse) -> CAM_lightBarInUse/1
  Seperate signals/5(CAM_publicVehicleType) -> CAM_publicVehicleType/1
  Seperate signals/4(CAM_vehicleType) -> CAM_vehicleType/1
  Seperate signals/3(CAM_vehicleID) -> CAM_vehicleID/1
  Seperate signals/2(CAM_messageID) -> CAM_messageID/1
  Seperate signals/1(CAM_warning) -> CAM_warning/1
  CAM_warning_in/1 -> Signal Matrix create/1(CAM_warning)
  CAM_messageID_in/1 -> Signal Matrix create/2(CAM_messageID)
  CAM_vehicleID_in/1 -> Signal Matrix create/3(CAM_vehicleID), Probe/1
  CAM_vehicleType_in/1 -> Signal Matrix create/4(CAM_vehicleType)
  CAM_publicVehicleType_in/1 -> Signal Matrix create/5(CAM_publicVehicleType)
  CAM_lightBarInUse_in/1 -> Signal Matrix create/6(CAM_lightBarInUse)
  CAM_sireneInUse_in/1 -> Signal Matrix create/7(CAM_sireneInUse)
  CAM_velocity_in/1 -> Signal Matrix create/8(CAM_velocity)
  CAM_acceleration_in/1 -> Signal Matrix create/9(CAM_acceleration)
  CAM_yawRate_in/1 -> Signal Matrix create/10(CAM_yawRate)
  CAM_turnAdvice_in/1 -> Signal Matrix create/11(CAM_turnAdvice)
  CAM_trafficLightPriority_in/1 -> Signal Matrix create/12(CAM_trafficLightPriority)
  CAM_GPSlat_in/1 -> Signal Matrix create/13(CAM_GPSlat)
  CAM_GPSlong_in/1 -> Signal Matrix create/14(CAM_GPSlong)
  CAM_GPSalt_in/1 -> Signal Matrix create/15(CAM_GPSalt)
  CAM_rotZ_in/1 -> Signal Matrix create/16(CAM_rotZ)
  Memory/1 -> For Iterator Subsystem/3(CAM_old)
  For Iterator Subsystem/1(CAM_o) -> Memory/1, Seperate signals/1(CAM)
  Probe/1 -> For Iterator Subsystem/2(Size)
  Signal Matrix create/1(CAM) -> CAM delay/1(in)
  MessageDelay/1 -> CAM delay/2(Tdelay)
  CAM delay/1(out) -> For Iterator Subsystem/1(CAM_in)
  For Iterator Subsystem/2(tmp_out) -> Memory1/1
  Memory1/1 -> For Iterator Subsystem/5(tmp_in)
  NoMissedMessages/1 -> Rounding Function1/1
  Rounding Function1/1 -> For Iterator Subsystem/4(NoMM)

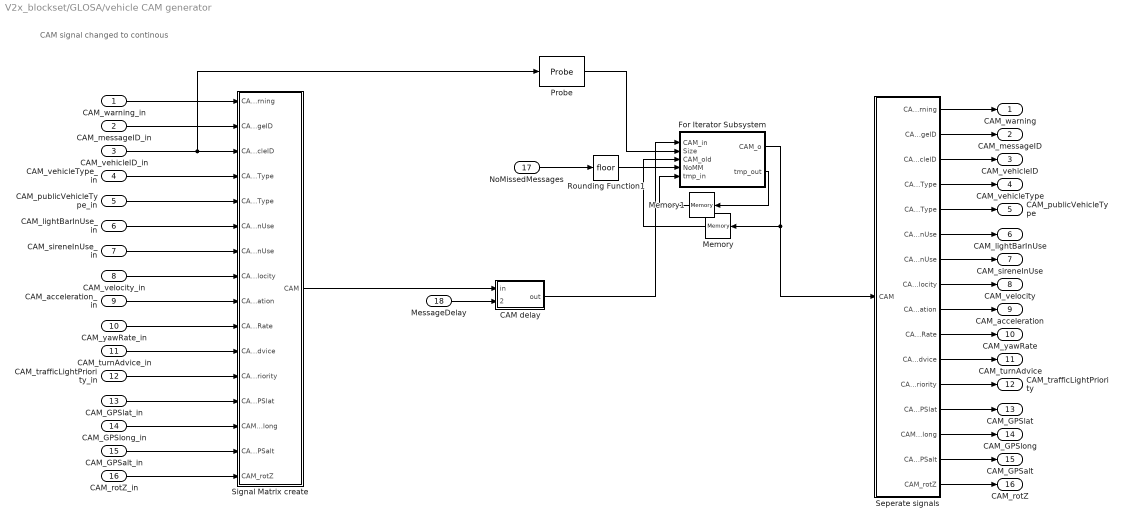
== system V2x_blockset/GLOSA/vehicle CAM generator ==
  note: CAM signal changed to continous
  CAM_warning_in : Inport
  CAM_messageID_in : Inport  Port=2
  CAM_vehicleID_in : Inport  Port=3
  CAM_vehicleType_in : Inport  Port=4
  CAM_publicVehicleType_in : Inport  Port=5
  CAM_lightBarInUse_in : Inport  Port=6
  CAM_sireneInUse_in : Inport  Port=7
  CAM_velocity_in : Inport  Port=8
  CAM_acceleration_in : Inport  Port=9
  CAM_yawRate_in : Inport  Port=10
  CAM_turnAdvice_in : Inport  Port=11
  CAM_trafficLightPriority_in : Inport  Port=12
  CAM_GPSlat_in : Inport  Port=13
  CAM_GPSlong_in : Inport  Port=14
  CAM_GPSalt_in : Inport  Port=15
  CAM_rotZ_in : Inport  Port=16
  NoMissedMessages : Inport  Port=17
  MessageDelay : Inport  Port=18
  CAM delay : Subsystem
  For Iterator Subsystem : Subsystem  TreatAsAtomicUnit=on
  Memory : Memory
  Memory1 : Memory
  Probe : Probe  ProbeWidth=off  ProbeSampleTime=off  ProbeComplexSignal=off  ProbeSignalDimensions=on
  Rounding Function1 : Rounding
  Seperate signals : Stateflow chart  TreatAsAtomicUnit=on
  Signal Matrix create : Stateflow chart  TreatAsAtomicUnit=on
  CAM_warning : Outport
  CAM_messageID : Outport  Port=2
  CAM_vehicleID : Outport  Port=3
  CAM_vehicleType : Outport  Port=4
  CAM_publicVehicleType : Outport  Port=5
  CAM_lightBarInUse : Outport  Port=6
  CAM_sireneInUse : Outport  Port=7
  CAM_velocity : Outport  Port=8
  CAM_acceleration : Outport  Port=9
  CAM_yawRate : Outport  Port=10
  CAM_turnAdvice : Outport  Port=11
  CAM_trafficLightPriority : Outport  Port=12
  CAM_GPSlat : Outport  Port=13
  CAM_GPSlong : Outport  Port=14
  CAM_GPSalt : Outport  Port=15
  CAM_rotZ : Outport  Port=16
  wires:
  Seperate signals/16(CAM_rotZ) -> CAM_rotZ/1
  Seperate signals/15(CAM_GPSalt) -> CAM_GPSalt/1
  Seperate signals/14(CAM_GPSlong) -> CAM_GPSlong/1
  Seperate signals/13(CAM_GPSlat) -> CAM_GPSlat/1
  Seperate signals/12(CAM_trafficLightPriority) -> CAM_trafficLightPriority/1
  Seperate signals/11(CAM_turnAdvice) -> CAM_turnAdvice/1
  Seperate signals/10(CAM_yawRate) -> CAM_yawRate/1
  Seperate signals/9(CAM_acceleration) -> CAM_acceleration/1
  Seperate signals/8(CAM_velocity) -> CAM_velocity/1
  Seperate signals/7(CAM_sireneInUse) -> CAM_sireneInUse/1
  Seperate signals/6(CAM_lightBarInUse) -> CAM_lightBarInUse/1
  Seperate signals/5(CAM_publicVehicleType) -> CAM_publicVehicleType/1
  Seperate signals/4(CAM_vehicleType) -> CAM_vehicleType/1
  Seperate signals/3(CAM_vehicleID) -> CAM_vehicleID/1
  Seperate signals/2(CAM_messageID) -> CAM_messageID/1
  Seperate signals/1(CAM_warning) -> CAM_warning/1
  CAM_warning_in/1 -> Signal Matrix create/1(CAM_warning)
  CAM_messageID_in/1 -> Signal Matrix create/2(CAM_messageID)
  CAM_vehicleID_in/1 -> Signal Matrix create/3(CAM_vehicleID), Probe/1
  CAM_vehicleType_in/1 -> Signal Matrix create/4(CAM_vehicleType)
  CAM_publicVehicleType_in/1 -> Signal Matrix create/5(CAM_publicVehicleType)
  CAM_lightBarInUse_in/1 -> Signal Matrix create/6(CAM_lightBarInUse)
  CAM_sireneInUse_in/1 -> Signal Matrix create/7(CAM_sireneInUse)
  CAM_velocity_in/1 -> Signal Matrix create/8(CAM_velocity)
  CAM_acceleration_in/1 -> Signal Matrix create/9(CAM_acceleration)
  CAM_yawRate_in/1 -> Signal Matrix create/10(CAM_yawRate)
  CAM_turnAdvice_in/1 -> Signal Matrix create/11(CAM_turnAdvice)
  CAM_trafficLightPriority_in/1 -> Signal Matrix create/12(CAM_trafficLightPriority)
  CAM_GPSlat_in/1 -> Signal Matrix create/13(CAM_GPSlat)
  CAM_GPSlong_in/1 -> Signal Matrix create/14(CAM_GPSlong)
  CAM_GPSalt_in/1 -> Signal Matrix create/15(CAM_GPSalt)
  CAM_rotZ_in/1 -> Signal Matrix create/16(CAM_rotZ)
  Memory/1 -> For Iterator Subsystem/3(CAM_old)
  For Iterator Subsystem/1(CAM_o) -> Memory/1, Seperate signals/1(CAM)
  Probe/1 -> For Iterator Subsystem/2(Size)
  Signal Matrix create/1(CAM) -> CAM delay/1(in)
  MessageDelay/1 -> CAM delay/2(Tdelay)
  CAM delay/1(out) -> For Iterator Subsystem/1(CAM_in)
  For Iterator Subsystem/2(tmp_out) -> Memory1/1
  Memory1/1 -> For Iterator Subsystem/5(tmp_in)
  NoMissedMessages/1 -> Rounding Function1/1
  Rounding Function1/1 -> For Iterator Subsystem/4(NoMM)

== system V2x_blockset/Rx_Noise/CAM delay ==
  in : Inport
  Tdelay : Inport  Port=2
  Bias : Bias  Bias=1
  Integer Delay{,1..9} (10 alike) : simulink/Discrete/Integer Delay  vinit=0.0  samptime=0.01  NumDelays=10
  Multiport Switch : MultiPortSwitch  Inputs=11  zeroidx=off
  Rounding Function : Rounding
  Saturation : Saturate  UpperLimit=11  LowerLimit=1
  out : Outport
  wires:
  Integer Delay9/1 -> Multiport Switch/12
  Saturation/1 -> Multiport Switch/1
  Bias/1 -> Saturation/1
  Rounding Function/1 -> Bias/1
  Tdelay/1 -> Rounding Function/1
  in/1 -> Integer Delay/1, Multiport Switch/2
  Integer Delay/1 -> Integer Delay1/1, Multiport Switch/3
  Integer Delay1/1 -> Integer Delay2/1, Multiport Switch/4
  Integer Delay2/1 -> Integer Delay3/1, Multiport Switch/5
  Integer Delay3/1 -> Integer Delay4/1, Multiport Switch/6
  Integer Delay4/1 -> Integer Delay5/1, Multiport Switch/7
  Integer Delay5/1 -> Integer Delay6/1, Multiport Switch/8
  Integer Delay6/1 -> Integer Delay7/1, Multiport Switch/9
  Integer Delay7/1 -> Integer Delay8/1, Multiport Switch/10
  Integer Delay8/1 -> Integer Delay9/1, Multiport Switch/11
  Multiport Switch/1 -> out/1

== system V2x_blockset/Rx_Noise/For Iterator Subsystem ==
  CAM_in : Inport
  Size : Inport  Port=2
  NoMM : Inport  Port=3
  tmp_in : Inport  Port=4
  Assignment1 : Assignment  NumberOfDimensions=2  IndexOptions=Index vector (port),Assign all  Indices=-1,-1  OutputSizes=2,16
  Assignment2 : Assignment  NumberOfDimensions=2  IndexOptions=Assign all,Index vector (port)  Indices=-1,-1  OutputSizes=2,16
  Embedded MATLAB Function : Stateflow chart  TreatAsAtomicUnit=on
  For Iterator : ForIterator  IterationSource=external
  Math Function : Math  Operator=transpose  SaturateOnIntegerOverflow=on
  Selector : Selector  NumberOfDimensions=2  InputPortWidth=3  IndexOptions=Select all,Index vector (dialog)  Indices=[1 3],1  OutputSizes=1,1
  Selector2 : Selector  NumberOfDimensions=2  InputPortWidth=3  IndexOptions=Index vector (port),Select all  Indices=1,1  OutputSizes=1,1
  Selector3 : Selector  IndexOptions=Index vector (port)  Indices=1  OutputSizes=1
  CAM_o : Outport
  tmp_out : Outport  Port=2
  wires:
  For Iterator/1 -> Assignment1/3, Assignment2/3, Selector3/2, Selector2/2, Embedded MATLAB Function/2(i)
  CAM_in/1 -> Assignment1/1, Embedded MATLAB Function/1(CAM), Selector/1
  Size/1 -> For Iterator/1
  NoMM/1 -> Embedded MATLAB Function/3(NoMM)
  tmp_in/1 -> Embedded MATLAB Function/4(tmp_in)
  Embedded MATLAB Function/2(tmp_out) -> Selector3/1
  Assignment1/1 -> CAM_o/1
  Selector/1 -> Math Function/1
  Math Function/1 -> Assignment2/1
  Assignment2/1 -> tmp_out/1
  Embedded MATLAB Function/1(CAM_o) -> Selector2/1
  Selector3/1 -> Assignment2/2
  Selector2/1 -> Assignment1/2

== system V2x_blockset/Traffic Controller/Intersection warning controller ==
  hostTurnAdvice : Inport
  hostRotZ : Inport  Port=2
  host GPS lat : Inport  Port=3
  host GPS long : Inport  Port=4
  host GPS alt : Inport  Port=5
  GPS lat : Inport  Port=6
  GPS long : Inport  Port=7
  GPS alt : Inport  Port=8
  actorID : Inport  Port=9
  targetVelocity : Inport  Port=10
  actorType : Inport  Port=11
  turnAdvice : Inport  Port=12
  rotZ : Inport  Port=13
  crossing detection range : Inport  Port=14
  Enabled Subsystem : Subsystem  TreatAsAtomicUnit=on
  Logical Operator : Logic  Operator=OR  Inputs=1  AllPortsSameDT=off  OutDataTypeStr=boolean
  Relational Operator : RelationalOperator  Operator===  OutDataTypeStr=boolean
  actorType crossing : Constant  Value=24
  actorType1 : InportShadow  Port=11
  warning left lane : Outport
  warning straight lane : Outport  Port=2
  warning right lane : Outport  Port=3
  wires:
  actorType crossing/1 -> Relational Operator/2
  Logical Operator/1 -> Enabled Subsystem/Enable
  Relational Operator/1 -> Logical Operator/1, Enabled Subsystem/1(crossingType)
  Enabled Subsystem/1(warning left lane) -> warning left lane/1
  Enabled Subsystem/2(warning straight lane) -> warning straight lane/1
  Enabled Subsystem/3(warning right lane) -> warning right lane/1
  actorType/1 -> Relational Operator/1
  hostTurnAdvice/1 -> Enabled Subsystem/2(hostTurnAdvice)
  hostRotZ/1 -> Enabled Subsystem/3(hostRotZ)
  host GPS lat/1 -> Enabled Subsystem/4(host GPS lat [deg])
  host GPS long/1 -> Enabled Subsystem/5(host GPS long [deg])
  host GPS alt/1 -> Enabled Subsystem/6(host GPS alt [m])
  GPS lat/1 -> Enabled Subsystem/7(GPS_lat)
  GPS long/1 -> Enabled Subsystem/8(GPS_long)
  GPS alt/1 -> Enabled Subsystem/9(GPS_alt)
  actorID/1 -> Enabled Subsystem/10(actorID)
  targetVelocity/1 -> Enabled Subsystem/11(targetVelocity)
  turnAdvice/1 -> Enabled Subsystem/12(turnAdvice)
  rotZ/1 -> Enabled Subsystem/13(rotZ)
  actorType1/1 -> Enabled Subsystem/14(actorType)
  crossing detection range/1 -> Enabled Subsystem/15(crossing detection range)

== system V2x_blockset/Traffic Controller/Road accident detection controller ==
  host_GPS lat [deg] : Inport
  host_GPS lat [deg]1 : Inport  Port=2
  host_GPS alt [m] : Inport  Port=3
  GPS lat [deg] : Inport  Port=4
  GPS long [deg] : Inport  Port=5
  GPS alt [deg] : Inport  Port=6
  warning : Inport  Port=7
  actorType : Inport  Port=8
  Compute distance to road accident : Subsystem
  Data Type Conversion2 : DataTypeConversion
  ITS road accident detection type ID : Constant  Value=25
  Logical Operator : Logic  Operator=OR  Inputs=1  AllPortsSameDT=off  OutDataTypeStr=boolean
  Logical Operator1 : Logic  AllPortsSameDT=off  OutDataTypeStr=boolean
  Logical Operator2 : Logic  Operator=OR  Inputs=4  AllPortsSameDT=off  OutDataTypeStr=boolean
  Relational Operator{,1..3} (4 alike) : RelationalOperator  Operator===  OutDataTypeStr=boolean
  buses or trucks ID : Constant  Value=3
  cars ID : Constant
  distance hold : Subsystem
  motors ID : Constant  Value=2
  warning hold : Subsystem
  RA_warning : Outport
  RA_distance : Outport  Port=2
  wires:
  Logical Operator1/1 -> Logical Operator/1, Compute distance to road accident/1(conditions)
  warning/1 -> Logical Operator1/1
  ITS road accident detection type ID/1 -> Relational Operator/2
  Compute distance to road accident/2(RA_distance) -> distance hold/1(dist)
  actorType/1 -> Relational Operator/1, Relational Operator1/1, Relational Operator2/1, Relational Operator3/1
  host_GPS lat [deg]/1 -> Compute distance to road accident/2(host_GPS lat [deg])
  host_GPS lat [deg]1/1 -> Compute distance to road accident/3(host_GPS lat [deg]1)
  host_GPS alt [m]/1 -> Compute distance to road accident/4(host_GPS alt [m])
  GPS lat [deg]/1 -> Compute distance to road accident/5(GPS lat [deg])
  GPS long [deg]/1 -> Compute distance to road accident/6(GPS long [deg])
  GPS alt [deg]/1 -> Compute distance to road accident/7(GPS alt [deg])
  Logical Operator/1 -> Compute distance to road accident/Enable
  Data Type Conversion2/1 -> warning hold/1(warn)
  Compute distance to road accident/1(RA_warning) -> Data Type Conversion2/1
  warning hold/1(warning) -> RA_warning/1
  distance hold/1(distance) -> RA_distance/1
  cars ID/1 -> Relational Operator1/2
  Relational Operator/1 -> Logical Operator2/1
  Relational Operator1/1 -> Logical Operator2/2
  Logical Operator2/1 -> Logical Operator1/2
  motors ID/1 -> Relational Operator2/2
  buses or trucks ID/1 -> Relational Operator3/2
  Relational Operator2/1 -> Logical Operator2/3
  Relational Operator3/1 -> Logical Operator2/4

== system V2x_blockset/Traffic Controller/Traffic signs and  traffic lights controller ==
  note: Traffic signs recognision
  hostRotZ : Inport
  hostVelocity : Inport  Port=2
  messageIDs : Inport  Port=3
  actorType : Inport  Port=4
  trafficLightPriority : Inport  Port=5
  rotZ : Inport  Port=6
  host GPS lat [deg] : Inport  Port=7
  host GPS long [deg] : Inport  Port=8
  host GPS alt [m] : Inport  Port=9
  GPS_lat : Inport  Port=10
  GPS_long : Inport  Port=11
  GPS_alt : Inport  Port=12
  Enabled Subsystem : Subsystem  TreatAsAtomicUnit=on
  Logical Operator : Logic  Operator=OR  Inputs=1  AllPortsSameDT=off  OutDataTypeStr=boolean
  Logical Operator1 : Logic  Operator=OR  AllPortsSameDT=off  OutDataTypeStr=boolean
  Relational Operator : RelationalOperator  Operator===  OutDataTypeStr=boolean
  Relational Operator1 : RelationalOperator  Operator===  OutDataTypeStr=boolean
  actorType traffic lights : Constant  Value=15
  actorType traffic sign : Constant  Value=14
  signsWarning : Outport
  signsMessage : Outport  Port=2
  lightsWarning : Outport  Port=3
  lightsMessage : Outport  Port=4
  lightsPriority : Outport  Port=5
  wires:
  GPS_alt/1 -> Enabled Subsystem/13(GPS_alt)
  GPS_long/1 -> Enabled Subsystem/12(GPS_long)
  GPS_lat/1 -> Enabled Subsystem/11(GPS_lat)
  host GPS alt [m]/1 -> Enabled Subsystem/10(host GPS alt [m])
  host GPS long [deg]/1 -> Enabled Subsystem/9(host GPS long [deg])
  host GPS lat [deg]/1 -> Enabled Subsystem/8(host GPS lat [deg])
  Enabled Subsystem/5(ligtsPriority) -> lightsPriority/1
  Enabled Subsystem/3(lightsWarning) -> lightsWarning/1
  Enabled Subsystem/4(ligtsMessage) -> lightsMessage/1
  Enabled Subsystem/1(signsWarning) -> signsWarning/1
  Enabled Subsystem/2(signsMessage) -> signsMessage/1
  trafficLightPriority/1 -> Enabled Subsystem/6(trafficLightPriority)
  Logical Operator1/1 -> Logical Operator/1
  Relational Operator1/1 -> Enabled Subsystem/2(trafficLightsType), Logical Operator1/2
  Relational Operator/1 -> Enabled Subsystem/1(trafficSignType), Logical Operator1/1
  actorType traffic lights/1 -> Relational Operator1/2
  hostRotZ/1 -> Enabled Subsystem/3(hostRotZ)
  rotZ/1 -> Enabled Subsystem/7(rotZ)
  messageIDs/1 -> Enabled Subsystem/5(messageID)
  hostVelocity/1 -> Enabled Subsystem/4(hostVelocity)
  Logical Operator/1 -> Enabled Subsystem/Enable
  actorType traffic sign/1 -> Relational Operator/2
  actorType/1 -> Relational Operator1/1, Relational Operator/1

== system V2x_blockset/signs CAM generator/Enabled Subsystem ==
  CAM_sig : Inport
  Enable : EnablePort  PropagateVarSize=During execution
  CAM_signals : Outport  OutputWhenDisabled=reset  InitialOutput=0
  wires:
  CAM_sig/1 -> CAM_signals/1

== system V2x_blockset/signs CAM generator/impulse generator1 ==
  CAM_time_step : Inport
  Add : Sum
  Compare To Zero : simulink/Logic and Bit Operations/Compare To Zero  SystemSampleTime=-1  relop=>  LogicOutDataTypeMode=uint8  ZeroCross=off
  Data Type Conversion : DataTypeConversion  OutDataTypeStr=boolean
  Detect Change : simulink/Logic and Bit Operations/Detect Change  SystemSampleTime=-1  vinit=0
  Digital Clock1 : DigitalClock  SampleTime=0.01
  Divide : Product  Inputs=*/
  Gain : Gain  Gain=pi
  Product : Product  RndMeth=Zero
  Trigonometric Function : Trigonometry
  constant : Constant
  experiment time step : Constant  Value=0.01  SampleTime=0
  enable : Outport
  wires:
  CAM_time_step/1 -> Divide/2
  Data Type Conversion/1 -> enable/1
  experiment time step/1 -> Add/2
  Add/1 -> Trigonometric Function/1
  Divide/1 -> Gain/1
  constant/1 -> Divide/1
  Product/1 -> Add/1
  Detect Change/1 -> Data Type Conversion/1
  Compare To Zero/1 -> Detect Change/1
  Trigonometric Function/1 -> Compare To Zero/1
  Gain/1 -> Product/2
  Digital Clock1/1 -> Product/1
